simulink model "pipeline_test"  (R2015a)
settings: Solver=ode23t  StartTime=0.0  StopTime=20e-3  RelTol=1e-4
libraries: fl_lib x6, nesl_utility x4, pipeline_lib x1
settings Model: Creator=tkw954  LastModifiedBy=tkw954
settings DebuggingCC: UnderspecifiedInitializationDetection=Classic  MergeDetectMultiDrivingBlocksExec=none  SolverPrmCheckMsg=warning  StateNameClashWarn=warning

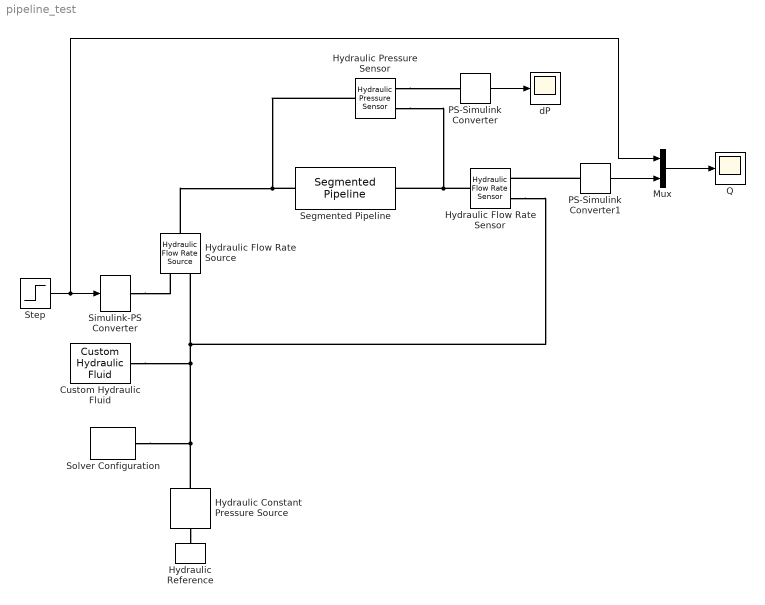
== system pipeline_test ==
  Custom Hydraulic Fluid : fl_lib/Hydraulic/Hydraulic Utilities/Custom Hydraulic Fluid  density=850 kg/m^3  viscosity_kin=18e-6 m^2/s  bulk=1e9 Pa  alpha=1e-5  range_error=2
  Hydraulic Constant Pressure Source : fl_lib/Hydraulic/Hydraulic Sources/Hydraulic Constant Pressure Source  commanded_pressure=10e6 Pa
  Hydraulic Flow Rate Sensor : fl_lib/Hydraulic/Hydraulic Sensors/Hydraulic Flow Rate Sensor
  Hydraulic Flow Rate Source : fl_lib/Hydraulic/Hydraulic Sources/Hydraulic Flow Rate Source
  Hydraulic Pressure Sensor : fl_lib/Hydraulic/Hydraulic Sensors/Hydraulic Pressure Sensor
  Hydraulic Reference : fl_lib/Hydraulic/Hydraulic Elements/Hydraulic Reference
  Mux : Mux  Inputs=2
  PS-Simulink Converter : nesl_utility/PS-Simulink Converter  PhysicalDomain=network_engine_domain  SubClassName=ps_output  LeftPortType=input  RightPortType=output  PseudoPeriodic=off  Frequencies=[]  Unit=1  AffineConversion=off
  PS-Simulink Converter1 : nesl_utility/PS-Simulink Converter  PhysicalDomain=network_engine_domain  SubClassName=ps_output  LeftPortType=input  RightPortType=output  PseudoPeriodic=off  Frequencies=[]  Unit=1  AffineConversion=off
  Q : Scope
      settings: YMin=-8.13152e-20  YMax=0.0013  SaveName=ScopeData2
  Segmented Pipeline : pipeline_lib/Segmented Pipeline  N=100  L=1  d=10e-3  e=1e-6  P0=10e6  Q0=0
  Simulink-PS Converter : nesl_utility/Simulink-PS Converter  PhysicalDomain=network_engine_domain  SubClassName=ps_input  LeftPortType=input  RightPortType=output  PseudoPeriodic=off  Frequencies=[]  NoiseDistribution=none  NoiseParameters=[]  Unit=1  AffineConversion=off  InputFiltering=off  SimscapeFilterOrder=1  InputFilterTimeConstant=0.001  UdotUserProvided=1
  Solver Configuration : nesl_utility/Solver Configuration  PhysicalDomain=network_engine_domain  SubClassName=solver  LeftPortType=input  RightPortType=generic  Accelerate=off  Tones=[]  Harmonics=[]  SimulateNoise=off  Profile=off  UseLocalSampling=off  EnableSwitchedLinearOptims=on  FrequencyDomain=off  UseCCode=off  RelTol=0.001  AbsTol=1e-06  MinStep=1e-09  ToWorkspace=off  RevertToSquareIcSolve=off  NumHomotopyIterations=100  DoDC=off  ResidualTolerance=1e-09  UseLocalSolver=off  LocalSolverChoice=NE_BACKWARD_EULER_ADVANCER  LocalSolverSampleTime=0.001  DoFixedCost=off  MaxNonlinIter=3  MaxModeIter=2  LinearAlgebra=Sparse  DelaysMemoryBudget=1024  AutomaticFiltering=on  FilteringTimeConstant=0.001
  Step : Step  Time=1e-3  After=30/60000  SampleTime=0
  dP : Scope
      settings: YMin=-1e+07  YMax=1e+07
  wires:
  Step/1 -> Simulink-PS Converter/1, Mux/1
  PS-Simulink Converter/1 -> dP/1
  PS-Simulink Converter1/1 -> Mux/2
  Mux/1 -> Q/1
  connections:
  Hydraulic Flow Rate Source/LConn1 -- Segmented Pipeline/LConn1 -- Hydraulic Pressure Sensor/LConn1
  Solver Configuration/RConn1 -- Hydraulic Constant Pressure Source/LConn1 -- Hydraulic Flow Rate Sensor/RConn2 -- Hydraulic Flow Rate Source/RConn2 -- Custom Hydraulic Fluid/RConn1
  Simulink-PS Converter/RConn1 -- Hydraulic Flow Rate Source/RConn1
  Hydraulic Pressure Sensor/RConn2 -- PS-Simulink Converter/LConn1
  Hydraulic Pressure Sensor/RConn1 -- Segmented Pipeline/RConn1 -- Hydraulic Flow Rate Sensor/LConn1
  PS-Simulink Converter1/LConn1 -- Hydraulic Flow Rate Sensor/RConn1
  Hydraulic Constant Pressure Source/RConn1 -- Hydraulic Reference/LConn1
